simulink model "gm_uz_pmsm_model_nonlinear_vnl"  (R2023a)
settings: Solver=FixedStepAuto  StartTime=0.0  StopTime=0.5  RelTol=1e-3
PreLoadFcn:
  | uz_pmsm_model_init_parameter
PostLoadFcn:
  | % Import the data from Excel for a lookup table
  | FluxMapData = readtable('C:\Users\Philipp\ultrazohm\ultrazohm_sw\ip_cores\uz_pmsm_model\FluxMapData_2023-05-26_13-07-57.csv');
  | % Row indices for lookup table
  | d_current_in_d_axis = FluxMapData(8:27,1:end);
  | % Column indices for lookup table
  | q_current_in_d_axis = FluxMapData(29:48,1:end);
  | % Output values for lookup table
  | d_Flux_d_axis = FluxMapData(50:69,1:end);
undefined symbols (not defined in the file or in its folder): d_current_d_Flux, d_current_q_Flux, Flux_d, Flux_q, friction_coefficient, inertia, k_i_d, k_p_d, k_p_q, L_d, L_q, Ldd, Ldq, Lqd, Lqq, polepair, psi_pm, q_current_d_Flux, q_current_q_Flux, R_1, setpoint_step, simulate_mechanical, simulate_open_loop, static_friction_torque, ts
libraries: hdlmdlgenlib x8, simulink x2, slpidlib x2
(part 1 of 2)
settings Model: Creator=ts  LastModifiedBy=Philipp
settings SolverCC: AlgebraicLoopSolver=TrustRegion  AutoInsertRateTranBlk=on
settings DataIOCC: LimitDataPoints=on  SaveOutput=off  SaveTime=off
settings OptimizationCC: BlockReduction=off  ConditionallyExecuteInputs=off  DefaultParameterBehavior=Inlined  LifeSpan=inf
settings DebuggingCC: AlgebraicLoopMsg=error  InheritedTsInSrcMsg=none  SingleTaskRateTransMsg=error  UnconnectedInputMsg=warning  UnconnectedOutputMsg=warning  UnconnectedLineMsg=warning  AllowSymbolicDim=off  StrictBusMsg=ErrorOnBusTreatedAsVector  SFUnexpectedBacktrackingDiag=warning  SFNoUnconditionalDefaultTransitionDiag=warning  SFExecutionAtInitializationDiag=none  ArithmeticOperatorsInVariantConditions=warning
settings HardwareCC: ProdBitPerPointer=32  ProdBitPerSizeT=32  ProdBitPerPtrDiffT=32  ProdLargestAtomicFloat=None  ProdIntDivRoundTo=Undefined  ProdEndianess=Unspecified  ProdWordSize=32  ProdHWDeviceType=ASIC/FPGA->ASIC/FPGA  ProdEqTarget=off
settings ModelReferenceCC: EnableRefExpFcnMdlSchedulingChecks=on
settings SFSimCC: SimUseLocalCustomCode=off  CustomCodeUndefinedFunction=UseInterfaceOnly
settings RTWCC: RTWUseLocalCustomCode=off  DLArmComputeVersion=19.05
settings CodeAppCC: StateflowObjectComments=on
settings GRTTargetCC: TargetLangStandard=C89/C90 (ANSI)
settings ConfigComp: CovScope=ReferencedModels  CovMetricSettings=dw  CovSaveCumulativeToWorkspaceVar=on  CovSaveSingleToWorkspaceVar=on  CovExternalEMLEnable=off  CovSFcnEnable=off

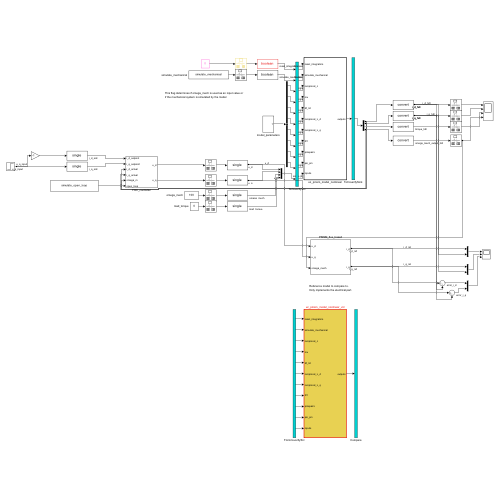
[thumbnail: Simulink's stored preview of the top-level diagram]
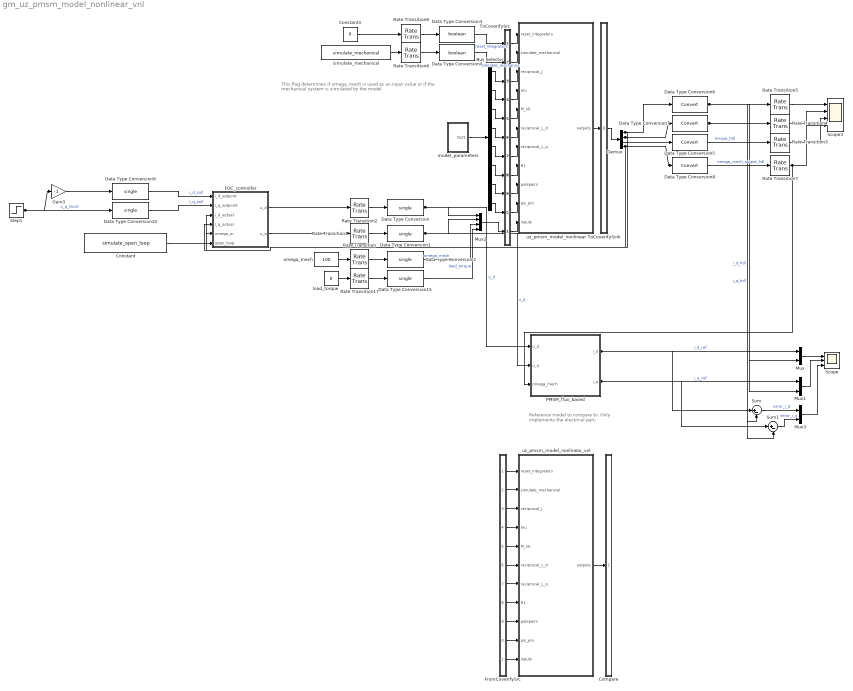
== system gm_uz_pmsm_model_nonlinear_vnl ==
  note: Reference model to compare to.
      | Only implements the electrical part.
  note: This flag determines if omega_mech is used as an input value or
      | if the mechanical system is simulated by the model
  Bus Selector : BusSelector  OutputSignals=1_J,mu,M_R0,1_L_d,1_L_q,R_1,polepair,psi_pm
  Compare : Subsystem
      mask Display: disp('')
  Constant : Constant  Value=simulate_open_loop
  Constant3 : Constant  Value=0
  Data Type Conversion{,1..2,9..10,15} (6 alike) : DataTypeConversion  OutDataTypeStr=single  SaturateOnIntegerOverflow=off  RndMeth=Floor
  Data Type Conversion3 : DataTypeConversion  OutDataTypeStr=boolean  SaturateOnIntegerOverflow=off  RndMeth=Floor
  Data Type Conversion4 : DataTypeConversion  OutDataTypeStr=boolean  SaturateOnIntegerOverflow=off  RndMeth=Floor
  Data Type Conversion{5..8} (4 alike) : DataTypeConversion  SaturateOnIntegerOverflow=off  RndMeth=Floor
  Demux : Demux
  FOC_controller : Subsystem
  FromCoverifySrc : Subsystem
      mask Display: disp('')
  Gain3 : Gain  Gain=-1
  Mux : Mux  Inputs=2
  Mux1 : Mux  Inputs=2
  Mux2 : Mux
  Mux3 : Mux  Inputs=2
  PMSM_flux_based : Subsystem
  Rate Transition{,1..2,6,8,17} (6 alike) : RateTransition  OutPortSampleTime=ts
  Rate Transition{3..5,7} (4 alike) : RateTransition
  Scope : Scope  NumInputPorts=3
  Scope3 : Scope  NumInputPorts=4
  Step1 : Step  Time=0.2  After=setpoint_step
  Sum : Sum  Inputs=|+-
  Sum1 : Sum  Inputs=|+-
  ToCoverifySink : Subsystem
      mask Display: disp('')
  ToCoverifySrc : Subsystem
      mask Display: disp('')
  load_torque : Constant  Value=0
  model_parameters : Subsystem
  omega_mech : Constant  Value=100
  simulate_mechanical : Constant  Value=simulate_mechanical
  uz_pmsm_model_nonlinear : Subsystem  TreatAsAtomicUnit=on
  uz_pmsm_model_nonlinear_vnl : Subsystem  TreatAsAtomicUnit=on
  wires:
  Rate Transition/1 -> Data Type Conversion2/1
  Rate Transition1/1 -> Data Type Conversion1/1
  Rate Transition2/1 -> Data Type Conversion/1
  Data Type Conversion6/1 -> Mux/2, Sum/2, Rate Transition5/1  "i_d_hdl"
  Data Type Conversion7/1 -> Rate Transition4/1, Mux1/2, Sum1/2  "i_q_hdl"
  Data Type Conversion5/1 -> Rate Transition3/1  "torque_hdl"
  Rate Transition4/1 -> Scope3/2
  Rate Transition5/1 -> Scope3/1
  Rate Transition3/1 -> Scope3/3
  Rate Transition6/1 -> Data Type Conversion3/1
  Constant3/1 -> Rate Transition6/1
  Rate Transition8/1 -> Data Type Conversion4/1
  simulate_mechanical/1 -> Rate Transition8/1
  load_torque/1 -> Rate Transition17/1
  Rate Transition17/1 -> Data Type Conversion15/1
  Mux/1 -> Scope/1
  Mux1/1 -> Scope/2
  PMSM_flux_based/2(i_q) -> Mux1/1, Sum1/1  "i_q_ref"
  PMSM_flux_based/1(i_d) -> Mux/1, Sum/1  "i_d_ref"
  Data Type Conversion8/1 -> Rate Transition7/1  "omega_mech_output_hdl"
  Rate Transition7/1 -> PMSM_flux_based/3(omega_mech), Scope3/4
  model_parameters/1(Out1) -> Bus Selector/1
  Sum/1 -> Mux3/1  "error_i_d"
  Sum1/1 -> Mux3/2  "error_i_q"
  Mux3/1 -> Scope/3
  Step1/1 -> Gain3/1, Data Type Conversion10/1  "u_q_input"
  Demux/3 -> Data Type Conversion5/1
  Gain3/1 -> Data Type Conversion9/1
  Demux/1 -> Data Type Conversion6/1, FOC_controller/3(i_d_actual)
  Demux/4 -> Data Type Conversion8/1, FOC_controller/5(omega_m)
  Demux/2 -> Data Type Conversion7/1, FOC_controller/4(i_q_actual)
  Data Type Conversion/1 -> PMSM_flux_based/1(u_d), Mux2/1  "u_d"
  Data Type Conversion1/1 -> PMSM_flux_based/2(u_q), Mux2/2  "u_q"
  Data Type Conversion15/1 -> Mux2/4  "load_torque"
  Data Type Conversion2/1 -> Mux2/3  "omega_mech"
  Data Type Conversion9/1 -> FOC_controller/1(i_d_setpont)  "i_d_soll"
  Data Type Conversion10/1 -> FOC_controller/2(i_q_setpoint)  "i_q_soll"
  FOC_controller/1(u_d) -> Rate Transition2/1
  FOC_controller/2(u_q) -> Rate Transition1/1
  omega_mech/1 -> Rate Transition/1
  Constant/1 -> FOC_controller/6(open_loop)
  ToCoverifySrc/1(out1) -> uz_pmsm_model_nonlinear/1(reset_integrators)
  ToCoverifySrc/2(out2) -> uz_pmsm_model_nonlinear/2(simulate_mechanical)
  ToCoverifySrc/3(out3) -> uz_pmsm_model_nonlinear/3(reciprocal_J)
  ToCoverifySrc/4(out4) -> uz_pmsm_model_nonlinear/4(mu)
  ToCoverifySrc/5(out5) -> uz_pmsm_model_nonlinear/5(M_n0)
  ToCoverifySrc/6(out6) -> uz_pmsm_model_nonlinear/6(reciprocal_L_d)
  ToCoverifySrc/7(out7) -> uz_pmsm_model_nonlinear/7(reciprocal_L_q)
  ToCoverifySrc/8(out8) -> uz_pmsm_model_nonlinear/8(R1)
  ToCoverifySrc/9(out9) -> uz_pmsm_model_nonlinear/9(polepairs)
  ToCoverifySrc/10(out10) -> uz_pmsm_model_nonlinear/10(psi_pm)
  ToCoverifySrc/11(out11) -> uz_pmsm_model_nonlinear/11(inputs)
  uz_pmsm_model_nonlinear/1(outputs) -> ToCoverifySink/1(in1)
  Data Type Conversion3/1 -> ToCoverifySrc/1(in1)  "reset_integrators"
  Data Type Conversion4/1 -> ToCoverifySrc/2(in2)  "simulate_mechanics"
  Bus Selector/1 -> ToCoverifySrc/3(in3)
  Bus Selector/2 -> ToCoverifySrc/4(in4)
  Bus Selector/3 -> ToCoverifySrc/5(in5)
  Bus Selector/4 -> ToCoverifySrc/6(in6)
  Bus Selector/5 -> ToCoverifySrc/7(in7)
  Bus Selector/6 -> ToCoverifySrc/8(in8)
  Bus Selector/7 -> ToCoverifySrc/9(in9)
  Bus Selector/8 -> ToCoverifySrc/10(in10)
  Mux2/1 -> ToCoverifySrc/11(in11)
  ToCoverifySink/1(out1) -> Demux/1
  FromCoverifySrc/1(out1) -> uz_pmsm_model_nonlinear_vnl/1(reset_integrators)
  FromCoverifySrc/2(out2) -> uz_pmsm_model_nonlinear_vnl/2(simulate_mechanical)
  FromCoverifySrc/3(out3) -> uz_pmsm_model_nonlinear_vnl/3(reciprocal_J)
  FromCoverifySrc/4(out4) -> uz_pmsm_model_nonlinear_vnl/4(mu)
  FromCoverifySrc/5(out5) -> uz_pmsm_model_nonlinear_vnl/5(M_n0)
  FromCoverifySrc/6(out6) -> uz_pmsm_model_nonlinear_vnl/6(reciprocal_L_d)
  FromCoverifySrc/7(out7) -> uz_pmsm_model_nonlinear_vnl/7(reciprocal_L_q)
  FromCoverifySrc/8(out8) -> uz_pmsm_model_nonlinear_vnl/8(R1)
  FromCoverifySrc/9(out9) -> uz_pmsm_model_nonlinear_vnl/9(polepairs)
  FromCoverifySrc/10(out10) -> uz_pmsm_model_nonlinear_vnl/10(psi_pm)
  FromCoverifySrc/11(out11) -> uz_pmsm_model_nonlinear_vnl/11(inputs)
  uz_pmsm_model_nonlinear_vnl/1(outputs) -> Compare/1(in1)

== system gm_uz_pmsm_model_nonlinear_vnl/Compare ==
  in1 : Inport
  Assert_outputs : Subsystem  mask{ToleranceValue=1e-07}
      settings: LibrarySourceBlock=hdlmdlgenlib/AssertRelEqIDC
  CleanupScopes : Subsystem
      settings: OpenFcn=|
      | blkName = gcb; %self block
      | idx = regexp(blkName, '/CleanupScopes$', 'once');
      | blkParent = blkName(1:idx-1);
      | blks=find_system(blkParent, 'LookUnderMasks', 'all','blocktype', 'Scope');
      | for itr = 1:length(blks)
      | 	 hScopeCfg = get_param(blks{itr},'ScopeConfiguration');
      | 	 hScopeCfg.Visible = ~ hScopeCfg.Visible;
      | end
      | drawnow;
      mask Display: fprintf(message('hdlcoder:cosim:vnl_dblclick').getString());
  Enable : Subsystem
      settings: OpenFcn=|
      | blkName = gcb;
      | idx = regexp(blkName, '/Enable$', 'once');
      | blkParent = blkName(1:idx-1);
      | blks=find_system(blkParent, 'LookUnderMasks', 'all','blocktype', 'Assertion');
      | e = get_param(blks{1}, 'Enabled');
      | if strcmp(e, 'on'), f= 'off';, else, f = 'on';, end
      | for ii=1:length(blks), set_param(blks{ii}, 'Enabled', f);, end
      | set_param(gcb, 'MaskDisplay',['fprintf(message(''hdlcoder:cosim:vnl_dblclick_assertions'',','''',upper(e),'''',').getString())']);
      mask Display: fprintf(message('hdlcoder:cosim:vnl_dblclick_assertions','OFF').getString());
  pathdelay1 : Delay  DelayLength=1
  wires:
  in1/1 -> pathdelay1/1
  pathdelay1/1 -> Assert_outputs/1(cosim)
  [out1] -> Assert_outputs/2(dut)

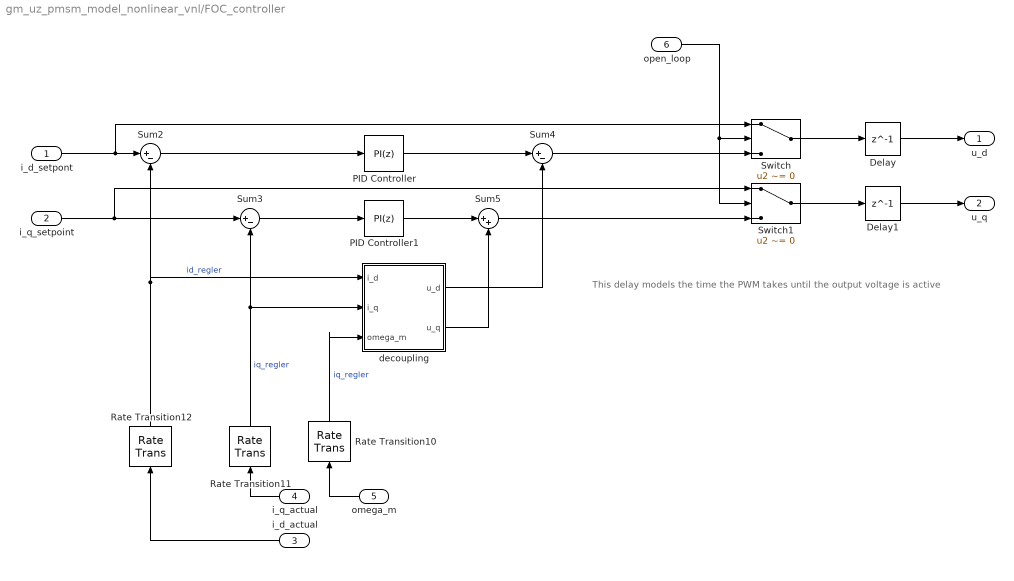
== system gm_uz_pmsm_model_nonlinear_vnl/FOC_controller ==
  note: This delay models the time the PWM takes until the output voltage is active
  i_d_setpont : Inport
  i_q_setpoint : Inport  Port=2
  i_d_actual : Inport  Port=3
  i_q_actual : Inport  Port=4
  omega_m : Inport  Port=5
  open_loop : Inport  Port=6
  Delay : Delay  DelayLength=1
  Delay1 : Delay  DelayLength=1
  PID Controller : slpidlib/PID Controller  Controller=PI  Form=Parallel  TimeDomain=Discrete-time  UseExternalTs=off  SampleTime=-1  IntegratorMethod=Forward Euler  FilterMethod=Forward Euler  ControllerParametersSource=internal  P=k_p_d  I=k_i_d  UseKiTs=off  D=0  N=100  UseFilter=on  TunerSelectOption=Transfer Function Based (PID Tuner App)  InitialConditionSource=internal  InitialConditionForIntegrator=0  InitialConditionForFilter=0  DifferentiatorICPrevScaledInput=0  ExternalReset=none  TrackingMode=off  Kt=1  LimitOutput=off  SatLimitsSource=internal  UpperSaturationLimit=inf  LowerSaturationLimit=-inf  LinearizeAsGain=on  AntiWindupMode=none  Kb=1  LimitIntegrator=off  UpperIntegratorSaturationLimit=inf  LowerIntegratorSaturationLimit=-inf  POutMin=[]  POutMax=[]  IOutMin=[]  IOutMax=[]  DOutMin=[]  DOutMax=[]  NOutMin=[]  NOutMax=[]  SumOutMin=[]  SumOutMax=[]  SaturationOutMin=[]  SaturationOutMax=[]  PParamMin=[]  PParamMax=[]  IParamMin=[]  IParamMax=[]  DParamMin=[]  DParamMax=[]  NParamMin=[]  NParamMax=[]  KbParamMin=[]  KbParamMax=[]  KtParamMin=[]  KtParamMax=[]  KbOutMin=[]  KbOutMax=[]  KtOutMin=[]  KtOutMax=[]  IntegratorOutMin=[]  IntegratorOutMax=[]  FilterOutMin=[]  FilterOutMax=[]  SumI1OutMin=[]  SumI1OutMax=[]  SumI2OutMin=[]  SumI2OutMax=[]  SumI3OutMin=[]  SumI3OutMax=[]  SumI4OutMin=[]  SumI4OutMax=[]  SumDOutMin=[]  SumDOutMax=[]  DifferentiatorOutMin=[]  DifferentiatorOutMax=[]  FilterDiffOutCoefMin=[]  FilterDiffOutCoefMax=[]  ReciprocalOutMin=[]  ReciprocalOutMax=[]  SumDenOutMin=[]  SumDenOutMax=[]  SumNumOutMin=[]  SumNumOutMax=[]  DivideOutMin=[]  DivideOutMax=[]  UdiffTsProdOutMin=[]  UdiffTsProdOutMax=[]  NTsProdOutMin=[]  NTsProdOutMax=[]  UintegralTsProdOutMin=[]  UintegralTsProdOutMax=[]  UngainTsProdOutMin=[]  UngainTsProdOutMax=[]  ClampingZeroOutDataTypeStr=Inherit: Inherit via back propagation  ClampingZeroOutMin=[]  ClampingZeroOutMax=[]  FilterDenConstantOutDataTypeStr=Inherit: Inherit via back propagation  FilterDenConstantOutMin=[]  FilterDenConstantOutMax=[]  PCopyOutDataTypeStr=Inherit: Inherit via back propagation  PCopyOutMin=[]  PCopyOutMax=[]  NCopyOutDataTypeStr=Inherit: Inherit via back propagation  NCopyOutMin=[]  NCopyOutMax=[]  IntegratorContinuousStateAttributes=''  IntegratorStateMustResolveToSignalObject=off  IntegratorRTWStateStorageClass=Auto  FilterContinuousStateAttributes=''  FilterStateMustResolveToSignalObject=off  FilterRTWStateStorageClass=Auto  ParallelPVariant=InternalParameters  IdealPVariant=Disabled  IVariant=InternalParameters  DVariant=Disabled  IntegratorVariant=Discrete  SatVariant=Disabled  AWVariant=Passthrough  PCopyVariant=Disabled  TRVariant=Disabled  FdbkBlocksVariant=Forward  IdealPFdbkVariant=Disabled  SatFdbkVariant=Disabled  DerivativeFilterVariant=Disabled  NVariant=Disabled  NCopyVariant=Disabled_SignalSpec  FilterICVariant=Disabled  IntegratorICVariant=InternalICs  ExternalResetVariant=Disabled  TRSumVariant=Passthrough  SumFdbkVariant=Disabled  SumVariant=Sum_PI  TsampFilterVariant=InternalTs  TsampNgainVariant=Passthrough  TsampIntegralVariant=Disabled_SignalSpec  ExternalSaturationOutDataTypeStr=Inherit: Same as second input
  PID Controller1 : slpidlib/PID Controller  Controller=PI  Form=Parallel  TimeDomain=Discrete-time  UseExternalTs=off  SampleTime=-1  IntegratorMethod=Forward Euler  FilterMethod=Forward Euler  ControllerParametersSource=internal  P=k_p_q  I=k_i_d  UseKiTs=off  D=0  N=100  UseFilter=on  TunerSelectOption=Transfer Function Based (PID Tuner App)  InitialConditionSource=internal  InitialConditionForIntegrator=0  InitialConditionForFilter=0  DifferentiatorICPrevScaledInput=0  ExternalReset=none  TrackingMode=off  Kt=1  LimitOutput=off  SatLimitsSource=internal  UpperSaturationLimit=inf  LowerSaturationLimit=-inf  LinearizeAsGain=on  AntiWindupMode=none  Kb=1  LimitIntegrator=off  UpperIntegratorSaturationLimit=inf  LowerIntegratorSaturationLimit=-inf  POutMin=[]  POutMax=[]  IOutMin=[]  IOutMax=[]  DOutMin=[]  DOutMax=[]  NOutMin=[]  NOutMax=[]  SumOutMin=[]  SumOutMax=[]  SaturationOutMin=[]  SaturationOutMax=[]  PParamMin=[]  PParamMax=[]  IParamMin=[]  IParamMax=[]  DParamMin=[]  DParamMax=[]  NParamMin=[]  NParamMax=[]  KbParamMin=[]  KbParamMax=[]  KtParamMin=[]  KtParamMax=[]  KbOutMin=[]  KbOutMax=[]  KtOutMin=[]  KtOutMax=[]  IntegratorOutMin=[]  IntegratorOutMax=[]  FilterOutMin=[]  FilterOutMax=[]  SumI1OutMin=[]  SumI1OutMax=[]  SumI2OutMin=[]  SumI2OutMax=[]  SumI3OutMin=[]  SumI3OutMax=[]  SumI4OutMin=[]  SumI4OutMax=[]  SumDOutMin=[]  SumDOutMax=[]  DifferentiatorOutMin=[]  DifferentiatorOutMax=[]  FilterDiffOutCoefMin=[]  FilterDiffOutCoefMax=[]  ReciprocalOutMin=[]  ReciprocalOutMax=[]  SumDenOutMin=[]  SumDenOutMax=[]  SumNumOutMin=[]  SumNumOutMax=[]  DivideOutMin=[]  DivideOutMax=[]  UdiffTsProdOutMin=[]  UdiffTsProdOutMax=[]  NTsProdOutMin=[]  NTsProdOutMax=[]  UintegralTsProdOutMin=[]  UintegralTsProdOutMax=[]  UngainTsProdOutMin=[]  UngainTsProdOutMax=[]  ClampingZeroOutDataTypeStr=Inherit: Inherit via back propagation  ClampingZeroOutMin=[]  ClampingZeroOutMax=[]  FilterDenConstantOutDataTypeStr=Inherit: Inherit via back propagation  FilterDenConstantOutMin=[]  FilterDenConstantOutMax=[]  PCopyOutDataTypeStr=Inherit: Inherit via back propagation  PCopyOutMin=[]  PCopyOutMax=[]  NCopyOutDataTypeStr=Inherit: Inherit via back propagation  NCopyOutMin=[]  NCopyOutMax=[]  IntegratorContinuousStateAttributes=''  IntegratorStateMustResolveToSignalObject=off  IntegratorRTWStateStorageClass=Auto  FilterContinuousStateAttributes=''  FilterStateMustResolveToSignalObject=off  FilterRTWStateStorageClass=Auto  ParallelPVariant=InternalParameters  IdealPVariant=Disabled  IVariant=InternalParameters  DVariant=Disabled  IntegratorVariant=Discrete  SatVariant=Disabled  AWVariant=Passthrough  PCopyVariant=Disabled  TRVariant=Disabled  FdbkBlocksVariant=Forward  IdealPFdbkVariant=Disabled  SatFdbkVariant=Disabled  DerivativeFilterVariant=Disabled  NVariant=Disabled  NCopyVariant=Disabled_SignalSpec  FilterICVariant=Disabled  IntegratorICVariant=InternalICs  ExternalResetVariant=Disabled  TRSumVariant=Passthrough  SumFdbkVariant=Disabled  SumVariant=Sum_PI  TsampFilterVariant=InternalTs  TsampNgainVariant=Passthrough  TsampIntegralVariant=Disabled_SignalSpec  ExternalSaturationOutDataTypeStr=Inherit: Same as second input
  Rate Transition10 : RateTransition  OutPortSampleTime=ts_regler
  Rate Transition11 : RateTransition  OutPortSampleTime=ts_regler
  Rate Transition12 : RateTransition  OutPortSampleTime=ts_regler
  Sum2 : Sum  Inputs=|+-
  Sum3 : Sum  Inputs=|+-
  Sum4 : Sum  Inputs=|+-
  Sum5 : Sum  Inputs=|++
  Switch : Switch  Criteria=u2 ~= 0  SaturateOnIntegerOverflow=off  InputSameDT=off
  Switch1 : Switch  Criteria=u2 ~= 0  SaturateOnIntegerOverflow=off  InputSameDT=off
  decoupling : Subsystem
  u_d : Outport
  u_q : Outport  Port=2
  wires:
  PID Controller/1 -> Sum4/1
  PID Controller1/1 -> Sum5/1
  Sum4/1 -> Switch/3
  i_d_actual/1 -> Rate Transition12/1
  i_d_setpont/1 -> Switch/1, Sum2/1
  Sum2/1 -> PID Controller/1
  Sum5/1 -> Switch1/3
  omega_m/1 -> Rate Transition10/1
  Sum3/1 -> PID Controller1/1
  i_q_actual/1 -> Rate Transition11/1
  Rate Transition12/1 -> decoupling/1(i_d), Sum2/2  "id_regler"
  Rate Transition11/1 -> decoupling/2(i_q), Sum3/2  "iq_regler"
  i_q_setpoint/1 -> Switch1/1, Sum3/1
  open_loop/1 -> Switch1/2, Switch/2
  Rate Transition10/1 -> decoupling/3(omega_m)  "iq_regler"
  decoupling/1(u_d) -> Sum4/2
  decoupling/2(u_q) -> Sum5/2
  Switch/1 -> Delay/1
  Switch1/1 -> Delay1/1
  Delay/1 -> u_d/1
  Delay1/1 -> u_q/1

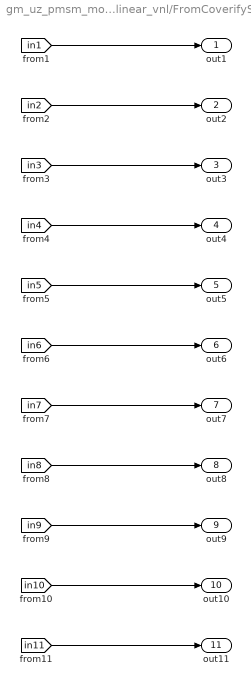
== system gm_uz_pmsm_model_nonlinear_vnl/FromCoverifySrc ==
  out1 : Outport
  out2 : Outport  Port=2
  out3 : Outport  Port=3
  out4 : Outport  Port=4
  out5 : Outport  Port=5
  out6 : Outport  Port=6
  out7 : Outport  Port=7
  out8 : Outport  Port=8
  out9 : Outport  Port=9
  out10 : Outport  Port=10
  out11 : Outport  Port=11
  wires:
  [in1] -> out1/1
  [in2] -> out2/1
  [in3] -> out3/1
  [in4] -> out4/1
  [in5] -> out5/1
  [in6] -> out6/1
  [in7] -> out7/1
  [in8] -> out8/1
  [in9] -> out9/1
  [in10] -> out10/1
  [in11] -> out11/1

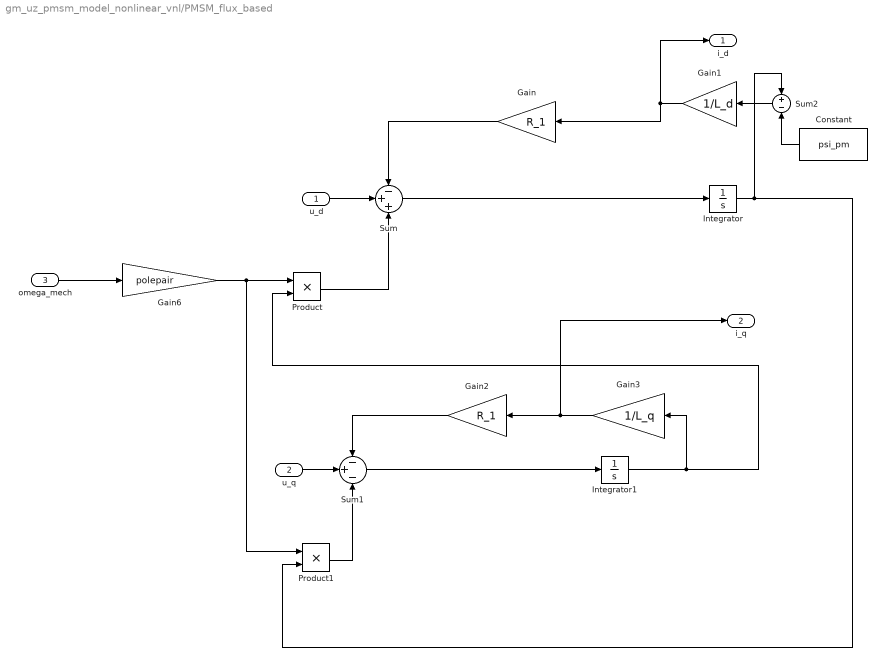
== system gm_uz_pmsm_model_nonlinear_vnl/PMSM_flux_based ==
  u_d : Inport
  u_q : Inport  Port=2
  omega_mech : Inport  Port=3
  Constant : Constant  Value=psi_pm
  Gain : Gain  Gain=R_1
  Gain1 : Gain  Gain=1/L_d
  Gain2 : Gain  Gain=R_1
  Gain3 : Gain  Gain=1/L_q
  Gain6 : Gain  Gain=polepair
  Integrator : Integrator
  Integrator1 : Integrator
  Product : Product
  Product1 : Product
  Sum : Sum  Inputs=-++
  Sum1 : Sum  Inputs=-+-
  Sum2 : Sum  Inputs=+-
  i_d : Outport
  i_q : Outport  Port=2
  wires:
  u_d/1 -> Sum/2
  u_q/1 -> Sum1/2
  Sum/1 -> Integrator/1
  Gain/1 -> Sum/1
  Integrator/1 -> Product1/2, Sum2/1
  Constant/1 -> Sum2/2
  Sum2/1 -> Gain1/1
  Gain1/1 -> Gain/1, i_d/1
  Gain6/1 -> Product1/1, Product/1
  Product/1 -> Sum/3
  Integrator1/1 -> Gain3/1, Product/2
  Product1/1 -> Sum1/3
  Sum1/1 -> Integrator1/1
  Gain2/1 -> Sum1/1
  Gain3/1 -> i_q/1, Gain2/1
  omega_mech/1 -> Gain6/1

== system gm_uz_pmsm_model_nonlinear_vnl/ToCoverifySink ==
  in1 : Inport
  out1 : Outport
  tag scope: out1=global
  wires:
  in1/1 -> out1/1, [out1]

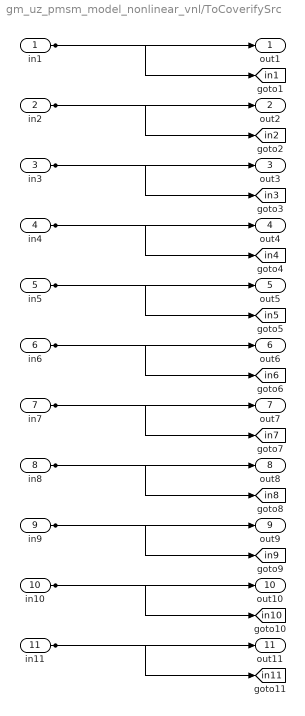
== system gm_uz_pmsm_model_nonlinear_vnl/ToCoverifySrc ==
  in1 : Inport
  in2 : Inport  Port=2
  in3 : Inport  Port=3
  in4 : Inport  Port=4
  in5 : Inport  Port=5
  in6 : Inport  Port=6
  in7 : Inport  Port=7
  in8 : Inport  Port=8
  in9 : Inport  Port=9
  in10 : Inport  Port=10
  in11 : Inport  Port=11
  out1 : Outport
  out2 : Outport  Port=2
  out3 : Outport  Port=3
  out4 : Outport  Port=4
  out5 : Outport  Port=5
  out6 : Outport  Port=6
  out7 : Outport  Port=7
  out8 : Outport  Port=8
  out9 : Outport  Port=9
  out10 : Outport  Port=10
  out11 : Outport  Port=11
  tag scope: in10=global, in11=global, in1=global, in2=global, in3=global, in4=global, in5=global, in6=global, in7=global, in8=global, in9=global
  wires:
  in1/1 -> out1/1, [in1]
  in2/1 -> out2/1, [in2]
  in3/1 -> out3/1, [in3]
  in4/1 -> out4/1, [in4]
  in5/1 -> out5/1, [in5]
  in6/1 -> out6/1, [in6]
  in7/1 -> out7/1, [in7]
  in8/1 -> out8/1, [in8]
  in9/1 -> out9/1, [in9]
  in10/1 -> out10/1, [in10]
  in11/1 -> out11/1, [in11]

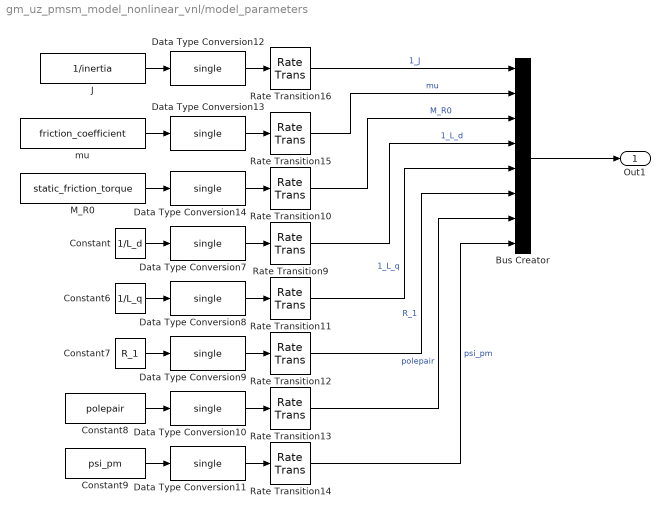
== system gm_uz_pmsm_model_nonlinear_vnl/model_parameters ==
  Bus Creator : BusCreator  Inputs=8
  Constant : Constant  Value=1/L_d
  Constant6 : Constant  Value=1/L_q
  Constant7 : Constant  Value=R_1
  Constant8 : Constant  Value=polepair
  Constant9 : Constant  Value=psi_pm
  Data Type Conversion{7..14} (8 alike) : DataTypeConversion  OutDataTypeStr=single  SaturateOnIntegerOverflow=off  RndMeth=Floor
  J : Constant  Value=1/inertia
  M_R0 : Constant  Value=static_friction_torque
  Rate Transition{9..16} (8 alike) : RateTransition  OutPortSampleTime=ts
  mu : Constant  Value=friction_coefficient
  Out1 : Outport
  wires:
  Data Type Conversion12/1 -> Rate Transition16/1
  Data Type Conversion7/1 -> Rate Transition9/1
  Rate Transition10/1 -> Bus Creator/3  "M_R0"
  Rate Transition14/1 -> Bus Creator/8  "psi_pm"
  Data Type Conversion14/1 -> Rate Transition10/1
  Rate Transition12/1 -> Bus Creator/6  "R_1"
  Rate Transition16/1 -> Bus Creator/1  "1_J"
  Rate Transition13/1 -> Bus Creator/7  "polepair"
  Bus Creator/1 -> Out1/1
  Data Type Conversion11/1 -> Rate Transition14/1
  Constant8/1 -> Data Type Conversion10/1
  Data Type Conversion9/1 -> Rate Transition12/1
  Rate Transition15/1 -> Bus Creator/2  "mu"
  Constant6/1 -> Data Type Conversion8/1
  Rate Transition9/1 -> Bus Creator/4  "1_L_d"
  J/1 -> Data Type Conversion12/1
  Data Type Conversion8/1 -> Rate Transition11/1
  Data Type Conversion10/1 -> Rate Transition13/1
  mu/1 -> Data Type Conversion13/1
  M_R0/1 -> Data Type Conversion14/1
  Rate Transition11/1 -> Bus Creator/5  "1_L_q"
  Data Type Conversion13/1 -> Rate Transition15/1
  Constant7/1 -> Data Type Conversion9/1
  Constant9/1 -> Data Type Conversion11/1
  Constant/1 -> Data Type Conversion7/1

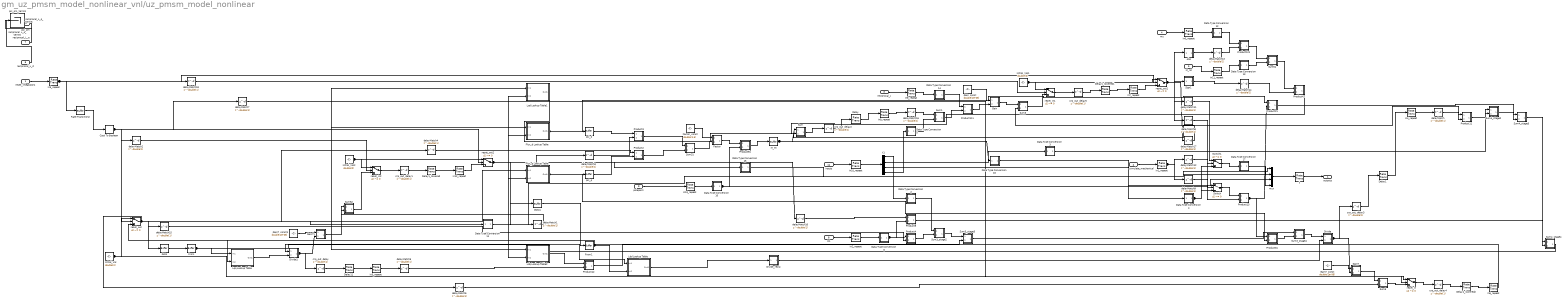
== system gm_uz_pmsm_model_nonlinear_vnl/uz_pmsm_model_nonlinear ==
  reset_integrators : Inport  OutDataTypeStr=boolean  PortDimensions=1  SampleTime=2e-06
  simulate_mechanical : Inport  Port=2  OutDataTypeStr=boolean  PortDimensions=1  SampleTime=2e-06
  reciprocal_J : Inport  Port=3  OutDataTypeStr=single  PortDimensions=1  SampleTime=2e-06
  mu : Inport  Port=4  OutDataTypeStr=single  PortDimensions=1  SampleTime=2e-06
  M_n0 : Inport  Port=5  OutDataTypeStr=single  PortDimensions=1  SampleTime=2e-06
  reciprocal_L_d : Inport  Port=6  OutDataTypeStr=single  PortDimensions=1  SampleTime=2e-06
  reciprocal_L_q : Inport  Port=7  OutDataTypeStr=single  PortDimensions=1  SampleTime=2e-06
  R1 : Inport  Port=8  OutDataTypeStr=single  PortDimensions=1  SampleTime=2e-06
  polepairs : Inport  Port=9  OutDataTypeStr=single  PortDimensions=1  SampleTime=2e-06
  psi_pm : Inport  Port=10  OutDataTypeStr=single  PortDimensions=1  SampleTime=2e-06
  inputs : Inport  Port=11  OutDataTypeStr=single  PortDimensions=[4]  SampleTime=2e-06
  Abs : Subsystem
      mask Display: disp('NFP\nabs');
  Cast To Boolean : DataTypeConversion  OutDataTypeStr=boolean
  Data Type Conversion10 : Subsystem
      mask Display: disp('NFP\nconv');
  Data Type Conversion11 : Subsystem
      mask Display: disp('NFP\nconv');
  Data Type Conversion12 : Subsystem
      mask Display: disp('NFP\nconv');
  Data Type Conversion13 : Subsystem
      mask Display: disp('NFP\nconv');
  Data Type Conversion14 : Subsystem
      mask Display: disp('NFP\nconv');
  Data Type Conversion15 : Subsystem
      mask Display: disp('NFP\nconv');
  Data Type Conversion16 : Subsystem
      mask Display: disp('NFP\nconv');
  Data Type Conversion17 : Subsystem
      mask Display: disp('NFP\nconv');
  Data Type Conversion2 : Subsystem
      mask Display: disp('NFP\nconv');
  Data Type Conversion3 : Subsystem
      mask Display: disp('NFP\nconv');
  Data Type Conversion4 : Subsystem
      mask Display: disp('NFP\nconv');
  Data Type Conversion5 : Subsystem
      mask Display: disp('NFP\nconv');
  Data Type Conversion6 : Subsystem
      mask Display: disp('NFP\nconv');
  Delay : RateTransition  OutPortSampleTimeOpt=Multiple of input port sample time  OutPortSampleTimeMultiple=200
  Delay1 : RateTransition  OutPortSampleTimeOpt=Multiple of input port sample time  OutPortSampleTimeMultiple=200
  Delay11 : RateTransition  OutPortSampleTimeOpt=Multiple of input port sample time  OutPortSampleTimeMultiple=200
  Delay1_lowered : RateTransition  OutPortSampleTimeOpt=Multiple of input port sample time  OutPortSampleTimeMultiple=200
  Delay1_lowered1 : RateTransition  OutPortSampleTimeOpt=Multiple of input port sample time  OutPortSampleTimeMultiple=200
  Delay1_lowered2 : RateTransition  OutPortSampleTimeOpt=Multiple of input port sample time  OutPortSampleTimeMultiple=200
  Divide : Subsystem
      mask Display: disp('NFP\nmul');
  Divide1 : Subsystem
      mask Display: disp('NFP\nmul');
  Divide_recip : Subsystem
      mask Display: disp('NFP\nmath');
  Factor : Subsystem
      mask Display: disp('NFP\nmul');
  Factor_const : Constant  Value=double(1.5)  OutDataTypeStr=double  SampleTime=1e-08
  Flux_d Lookup Table : Subsystem
  Flux_q Lookup Table : Subsystem
  From : hdlmdlgenlib/Buffer
  From1 : hdlmdlgenlib/Buffer
  Gain : Subsystem
      mask Display: disp('NFP\nmul');
  Gain7 : Subsystem
      mask Display: disp('NFP\nmul');
  Gain71 : Subsystem
      mask Display: disp('NFP\nmul');
  Gain7_const : Constant  Value=double(2e-06)  OutDataTypeStr=double  SampleTime=1e-08
  Gain7_const1 : Constant  Value=double(2e-06)  OutDataTypeStr=double  SampleTime=1e-08
  Gain_const : Constant  Value=double(2e-06)  OutDataTypeStr=double  SampleTime=1e-08
  Goto : hdlmdlgenlib/Buffer
  Goto1 : hdlmdlgenlib/Buffer
  Initial_Val : Constant  Value=double(0)  OutDataTypeStr=double  SampleTime=1e-08
  Initial_Val1 : Constant  Value=double(0)  OutDataTypeStr=double  SampleTime=1e-08
  Initial_Val2 : Constant  Value=double(0)  OutDataTypeStr=double  SampleTime=1e-08
  Ldd Lookup Table : Subsystem
  Ldq Lookup Table2 : Subsystem
  Lqd Lookup Table1 : Subsystem
  Lqq Lookup Table : Subsystem
  M_Mi : hdlmdlgenlib/Buffer
  Product11 : Subsystem
      mask Display: disp('NFP\nmul');
  Product111 : Subsystem
      mask Display: disp('NFP\nmul');
  Product12 : Subsystem
      mask Display: disp('NFP\nmul');
  Product121 : Subsystem
      mask Display: disp('NFP\nmul');
  Product13 : Subsystem
      mask Display: disp('NFP\nmul');
  Product2 : Subsystem
      mask Display: disp('NFP\nmul');
  Product21 : Subsystem
      mask Display: disp('NFP\nmul');
  Product3 : Subsystem
      mask Display: disp('NFP\nmul');
  Product31 : Subsystem
      mask Display: disp('NFP\nmul');
  Product4 : Subsystem
      mask Display: disp('NFP\nmul');
  Product41 : Subsystem
      mask Display: disp('NFP\nmul');
  Product9 : Subsystem
      mask Display: disp('NFP\nmul');
  Product91 : Subsystem
      mask Display: disp('NFP\nmul');
  Rate Transition2 : hdlmdlgenlib/Buffer
  Sign1 : Subsystem
      mask Display: disp('NFP\nsignum');
  Sum : Subsystem
      mask Display: disp('NFP\nadd');
  Sum1 : Subsystem
      mask Display: disp('NFP\nadd');
  Sum3 : Subsystem
      mask Display: disp('NFP\nadd');
  Sum31 : Subsystem
      mask Display: disp('NFP\nadd');
  Sum3_stage2 : Subsystem
      mask Display: disp('NFP\nadd');
  Sum3_stage3 : Subsystem
      mask Display: disp('NFP\nadd');
  Sum3_stage4 : Subsystem
      mask Display: disp('NFP\nadd');
  Sum4_stage2 : Subsystem
      mask Display: disp('NFP\nadd');
  Sum4_stage3 : Subsystem
      mask Display: disp('NFP\nadd');
  Sum4_stage4 : Subsystem
      mask Display: disp('NFP\nadd');
  Sum5 : Subsystem
      mask Display: disp('NFP\nadd');
  Sum51 : Subsystem
      mask Display: disp('NFP\nadd');
  Sum52 : Subsystem
      mask Display: disp('NFP\nadd');
  Switch : Switch  Criteria=u2 ~= 0  Threshold=double(0)  OutDataTypeStr=double  SampleTime=1e-08  SaturateOnIntegerOverflow=off  InputSameDT=off
  Switch1 : Switch  Criteria=u2 ~= 0  Threshold=double(0)  OutDataTypeStr=double  SampleTime=1e-08  SaturateOnIntegerOverflow=off  InputSameDT=off
  crp_out_delay{,1..5} (6 alike) : Delay  DelayLength=double(1)  InitialCondition=0  SampleTime=1e-08
  delayMatch{,1..18} (19 alike) : Delay  DelayLength=double(1)  InitialCondition=0  SampleTime=1e-08
  in0_repeat : RateTransition  Integrity=off  Deterministic=off  OutPortSampleTimeOpt=Multiple of input port sample time  OutPortSampleTimeMultiple=1/200
  in10_repeat : RateTransition  Integrity=off  Deterministic=off  OutPortSampleTimeOpt=Multiple of input port sample time  OutPortSampleTimeMultiple=1/200
  in11_repeat : RateTransition  Integrity=off  Deterministic=off  OutPortSampleTimeOpt=Multiple of input port sample time  OutPortSampleTimeMultiple=1/200
  in12_repeat : RateTransition  Integrity=off  Deterministic=off  OutPortSampleTimeOpt=Multiple of input port sample time  OutPortSampleTimeMultiple=1/200
  in13_repeat : RateTransition  Integrity=off  Deterministic=off  OutPortSampleTimeOpt=Multiple of input port sample time  OutPortSampleTimeMultiple=1/200
  in1_repeat : RateTransition  Integrity=off  Deterministic=off  OutPortSampleTimeOpt=Multiple of input port sample time  OutPortSampleTimeMultiple=1/200
  in2_repeat : RateTransition  Integrity=off  Deterministic=off  OutPortSampleTimeOpt=Multiple of input port sample time  OutPortSampleTimeMultiple=1/200
  in3_repeat : RateTransition  Integrity=off  Deterministic=off  OutPortSampleTimeOpt=Multiple of input port sample time  OutPortSampleTimeMultiple=1/200
  in4_repeat : RateTransition  Integrity=off  Deterministic=off  OutPortSampleTimeOpt=Multiple of input port sample time  OutPortSampleTimeMultiple=1/200
  in5_repeat : RateTransition  Integrity=off  Deterministic=off  OutPortSampleTimeOpt=Multiple of input port sample time  OutPortSampleTimeMultiple=1/200
  in6_repeat : RateTransition  Integrity=off  Deterministic=off  OutPortSampleTimeOpt=Multiple of input port sample time  OutPortSampleTimeMultiple=1/200
  in7_repeat : RateTransition  Integrity=off  Deterministic=off  OutPortSampleTimeOpt=Multiple of input port sample time  OutPortSampleTimeMultiple=1/200
  in8_repeat : RateTransition  Integrity=off  Deterministic=off  OutPortSampleTimeOpt=Multiple of input port sample time  OutPortSampleTimeMultiple=1/200
  in9_repeat : RateTransition  Integrity=off  Deterministic=off  OutPortSampleTimeOpt=Multiple of input port sample time  OutPortSampleTimeMultiple=1/200
  mux : Mux
  psi_d : hdlmdlgenlib/Buffer
  psi_pm_term9 : Terminator
  psi_q : hdlmdlgenlib/Buffer
  reciprocal_L_d_term5 : Terminator
  reciprocal_L_q_term6 : Terminator
  reset_in : Switch  Criteria=u2 ~= 0  Threshold=double(0)  OutDataTypeStr=double  SampleTime=1e-08  SaturateOnIntegerOverflow=off  InputSameDT=off
  reset_in1 : Switch  Criteria=u2 ~= 0  Threshold=double(0)  OutDataTypeStr=double  SampleTime=1e-08  SaturateOnIntegerOverflow=off  InputSameDT=off
  reset_in2 : Switch  Criteria=u2 ~= 0  Threshold=double(0)  OutDataTypeStr=double  SampleTime=1e-08  SaturateOnIntegerOverflow=off  InputSameDT=off
  reset_out : Switch  Criteria=u2 ~= 0  Threshold=double(0)  OutDataTypeStr=double  SampleTime=1e-08  SaturateOnIntegerOverflow=off  InputSameDT=off
  reset_out1 : Switch  Criteria=u2 ~= 0  Threshold=double(0)  OutDataTypeStr=double  SampleTime=1e-08  SaturateOnIntegerOverflow=off  InputSameDT=off
  reset_out2 : Switch  Criteria=u2 ~= 0  Threshold=double(0)  OutDataTypeStr=double  SampleTime=1e-08  SaturateOnIntegerOverflow=off  InputSameDT=off
  t : RateTransition  OutPortSampleTimeOpt=Multiple of input port sample time  OutPortSampleTimeMultiple=200
  t1 : Demux
  outputs : Outport  SampleTime=2e-06
  wires:
  reset_out1/1 -> delayMatch8/1, delayMatch11/1, Sign1/1(In1), Abs/1(In1), delayMatch17/1
  delayMatch7/1 -> reset_in/2
  delayMatch6/1 -> Sum5/2(In2)
  delayMatch2/1 -> reset_in2/2
  delayMatch1/1 -> Sum52/2(In2)
  delayMatch12/1 -> Switch1/2
  delayMatch11/1 -> Switch1/1
  Gain71/1(Out1) -> Sum52/1(In1)
  Gain/1(Out1) -> Sum3/1(In1)
  Gain7/1(Out1) -> Sum5/1(In1)
  Data Type Conversion10/1(Out1) -> Product91/2(In2), Product13/2(In2)
  Product13/1(Out1) -> Product31/1(In1), Product21/2(In2)
  Sum4_stage4/1(Out1) -> Divide1/1(In1)
  Sum4_stage3/1(Out1) -> Sum4_stage4/1(In1)
  Sum4_stage2/1(Out1) -> Sum4_stage3/1(In1)
  Sum52/1(Out1) -> reset_in2/3
  Data Type Conversion11/1(Out1) -> mux/1
  Product2/1(Out1) -> Sum31/2(In2)
  Sum31/1(Out1) -> Factor/2(In2)
  Sum/1(Out1) -> crp_out_delay2/1
  Product41/1(Out1) -> Sum/2(In2)
  Sum51/1(Out1) -> Product41/1(In1)
  Data Type Conversion13/1(Out1) -> Sum51/2(In2)
  Product121/1(Out1) -> Sum51/1(In1)
  Abs/1(Out1) -> delayMatch13/1
  Sign1/1(Out1) -> delayMatch14/1
  Sum1/1(Out1) -> Product111/2(In2)
  Product111/1(Out1) -> Gain/2(In2)
  Data Type Conversion14/1(Out1) -> Product111/1(In1)
  Sum3/1(Out1) -> reset_in1/3
  Sum3_stage4/1(Out1) -> Divide/1(In1)
  Sum3_stage3/1(Out1) -> Sum3_stage4/1(In1)
  Sum3_stage2/1(Out1) -> Sum3_stage3/1(In1)
  Divide_recip/1(Out1) -> Divide/2(In2)
  Sum5/1(Out1) -> reset_in/3
  Product11/1(Out1) -> Sum4_stage2/2(In2)
  Product12/1(Out1) -> Sum3_stage3/2(In2)
  Product3/1(Out1) -> Sum31/1(In1)
  Product4/1(Out1) -> Sum3_stage2/2(In2)
  Data Type Conversion6/1(Out1) -> Product9/2(In2), Product4/1(In1)
  Product9/1(Out1) -> Sum4_stage4/2(In2)
  Data Type Conversion12/1(Out1) -> Product121/1(In1)
  Cast To Boolean/1 -> reset_out/2, reset_out2/2, delayMatch2/1, delayMatch7/1
  reset_out/1 -> delayMatch4/1, Data Type Conversion11/1(In1), Lqd Lookup Table1/1(In1), Ldq Lookup Table2/1(In1), Flux_q Lookup Table/1(In1), Flux_d Lookup Table/1(In1), Goto/1, delayMatch15/1, delayMatch6/1
  reset_out2/1 -> delayMatch3/1, Data Type Conversion15/1(In1), Lqd Lookup Table1/2(In2), Ldq Lookup Table2/2(In2), Flux_q Lookup Table/2(In2), Flux_d Lookup Table/2(In2), Goto1/1, delayMatch10/1, delayMatch1/1
  delayMatch16/1 -> Sum1/1(In1)
  delayMatch18/1 -> reset_in1/2
  delayMatch9/1 -> Switch/2
  Gain7_const1/1 -> Gain71/1(In1)
  Factor_const/1 -> Factor/1(In1)
  Gain_const/1 -> Gain/1(In1)
  Gain7_const/1 -> Gain7/1(In1)
  delayMatch/1 -> Product11/1(In1)
  delayMatch5/1 -> Product12/2(In2)
  Product21/1(Out1) -> Sum4_stage3/2(In2)
  Divide1/1(Out1) -> crp_out_delay/1, Gain71/2(In2)
  reset_in2/1 -> crp_out_delay1/1
  Initial_Val2/1 -> reset_in2/1, reset_out2/1
  delayMatch10/1 -> Product9/1(In1)
  delayMatch3/1 -> Product3/2(In2)
  Data Type Conversion15/1(Out1) -> mux/2
  delayMatch4/1 -> Product2/1(In1)
  Factor/1(Out1) -> Product91/1(In1)
  Product91/1(Out1) -> M_Mi/1
  M_Mi/1 -> Data Type Conversion16/1(In1), Sum/1(In1)
  delayMatch13/1 -> Product121/2(In2)
  delayMatch14/1 -> Product41/2(In2)
  delayMatch8/1 -> Switch/1
  Switch/1 -> Product13/1(In1)
  Data Type Conversion4/1(Out1) -> Switch1/3, Switch/3
  t1/4 -> Data Type Conversion5/1(In1)
  t1/3 -> Data Type Conversion4/1(In1)
  t1/2 -> Data Type Conversion3/1(In1)
  t1/1 -> Data Type Conversion2/1(In1)
  Data Type Conversion5/1(Out1) -> Sum1/2(In2)
  reset_in1/1 -> crp_out_delay5/1
  Initial_Val1/1 -> reset_in1/1, reset_out1/1
  delayMatch17/1 -> Sum3/2(In2)
  Data Type Conversion3/1(Out1) -> Sum4_stage2/1(In1)
  Data Type Conversion2/1(Out1) -> Sum3_stage2/1(In1)
  Divide/1(Out1) -> crp_out_delay3/1, Gain7/2(In2)
  reset_in/1 -> crp_out_delay4/1
  Initial_Val/1 -> reset_in/1, reset_out/1
  Rate Transition2/1 -> Cast To Boolean/1
  delayMatch15/1 -> Product4/2(In2)
  Lqd Lookup Table1/1(Out1) -> Product11/2(In2)
  Ldq Lookup Table2/1(Out1) -> Product12/1(In1)
  Flux_q Lookup Table/1(Out1) -> psi_q/1, Product31/2(In2)
  Product31/1(Out1) -> Sum3_stage4/2(In2)
  psi_q/1 -> Product2/2(In2)
  Flux_d Lookup Table/1(Out1) -> psi_d/1, Product21/1(In1)
  psi_d/1 -> Product3/1(In1)
  Goto/1 -> From/1
  From/1 -> Lqq Lookup Table/1(In1), Ldd Lookup Table/1(In1)
  Ldd Lookup Table/1(Out1) -> Divide_recip/1(In1)
  From1/1 -> Lqq Lookup Table/2(In2), Ldd Lookup Table/2(In2)
  Goto1/1 -> From1/1
  Lqq Lookup Table/1(Out1) -> Divide1/2(In2)
  Switch1/1 -> Data Type Conversion17/1(In1)
  Data Type Conversion17/1(Out1) -> mux/4
  Data Type Conversion16/1(Out1) -> mux/3
  crp_out_delay5/1 -> Delay1_lowered1/1
  crp_out_delay4/1 -> Delay1_lowered2/1
  crp_out_delay3/1 -> Delay1/1
  crp_out_delay2/1 -> Delay/1
  crp_out_delay1/1 -> Delay1_lowered/1
  crp_out_delay/1 -> Delay11/1
  in3_repeat/1 -> delayMatch5/1
  Delay11/1 -> in3_repeat/1
  in4_repeat/1 -> delayMatch/1
  Delay1/1 -> in4_repeat/1
  in6_repeat/1 -> reset_out/3
  Delay1_lowered2/1 -> in6_repeat/1
  in7_repeat/1 -> reset_out1/3
  Delay1_lowered1/1 -> in7_repeat/1
  in9_repeat/1 -> delayMatch16/1
  Delay/1 -> in9_repeat/1
  in12_repeat/1 -> reset_out2/3
  Delay1_lowered/1 -> in12_repeat/1
  mux/1 -> t/1
  in13_repeat/1 -> Data Type Conversion10/1(In1)
  in11_repeat/1 -> Data Type Conversion13/1(In1)
  in10_repeat/1 -> t1/1
  in8_repeat/1 -> Data Type Conversion14/1(In1)
  in5_repeat/1 -> reset_out1/2, Rate Transition2/1, delayMatch18/1
  in2_repeat/1 -> Data Type Conversion6/1(In1)
  in1_repeat/1 -> delayMatch9/1, delayMatch12/1
  in0_repeat/1 -> Data Type Conversion12/1(In1)
  t/1 -> outputs/1
  inputs/1 -> in10_repeat/1
  psi_pm/1 -> psi_pm_term9/1
  polepairs/1 -> in13_repeat/1
  R1/1 -> in2_repeat/1
  reciprocal_L_q/1 -> reciprocal_L_q_term6/1
  reciprocal_L_d/1 -> reciprocal_L_d_term5/1
  M_n0/1 -> in11_repeat/1
  mu/1 -> in0_repeat/1
  reciprocal_J/1 -> in8_repeat/1
  simulate_mechanical/1 -> in1_repeat/1
  reset_integrators/1 -> in5_repeat/1

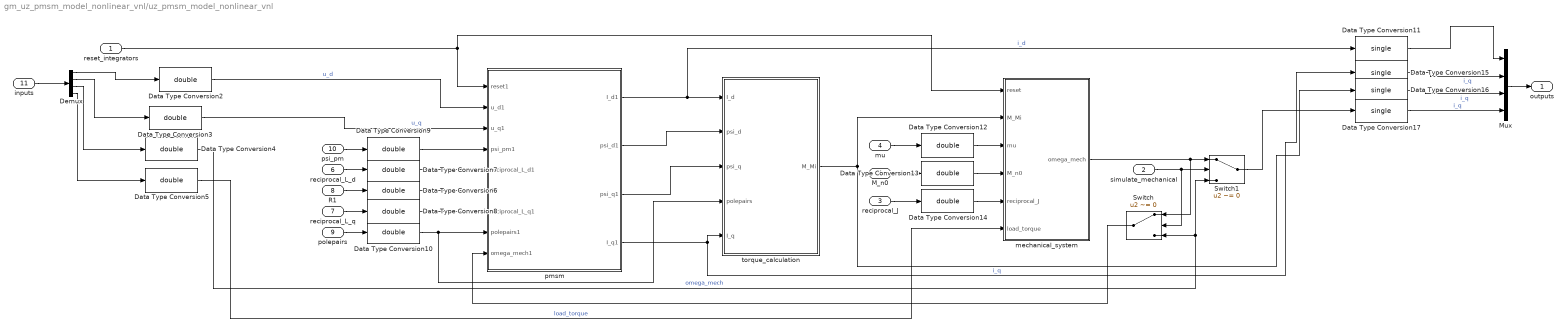
== system gm_uz_pmsm_model_nonlinear_vnl/uz_pmsm_model_nonlinear_vnl ==
  reset_integrators : Inport
  simulate_mechanical : Inport  Port=2
  reciprocal_J : Inport  Port=3
  mu : Inport  Port=4
  M_n0 : Inport  Port=5
  reciprocal_L_d : Inport  Port=6
  reciprocal_L_q : Inport  Port=7
  R1 : Inport  Port=8
  polepairs : Inport  Port=9
  psi_pm : Inport  Port=10
  inputs : Inport  Port=11
  Data Type Conversion{2..10,12..14} (12 alike) : DataTypeConversion  OutDataTypeStr=double  RndMeth=Nearest  SaturateOnIntegerOverflow=off
  Data Type Conversion{11,15..17} (4 alike) : DataTypeConversion  OutDataTypeStr=single  RndMeth=Nearest  SaturateOnIntegerOverflow=off
  Demux : Demux
  Mux : Mux
  Switch : Switch  Criteria=u2 ~= 0  SaturateOnIntegerOverflow=off  InputSameDT=off
  Switch1 : Switch  Criteria=u2 ~= 0  SaturateOnIntegerOverflow=off  InputSameDT=off
  mechanical_system : Subsystem
  pmsm : Subsystem
  torque_calculation : Subsystem
  outputs : Outport
  wires:
  Mux/1 -> outputs/1
  inputs/1 -> Demux/1
  Demux/4 -> Data Type Conversion5/1
  Demux/3 -> Data Type Conversion4/1
  Demux/2 -> Data Type Conversion3/1
  Demux/1 -> Data Type Conversion2/1
  Data Type Conversion11/1 -> Mux/1
  Data Type Conversion15/1 -> Mux/2  "i_q"
  Data Type Conversion16/1 -> Mux/3  "i_q"
  Data Type Conversion17/1 -> Mux/4  "i_q"
  pmsm/1(I_d1) -> torque_calculation/1(I_d), Data Type Conversion11/1  "i_d"
  pmsm/4(I_q1) -> Data Type Conversion15/1, torque_calculation/5(I_q)  "i_q"
  mechanical_system/1(omega_mech) -> Switch1/1, Switch/1
  Data Type Conversion3/1 -> pmsm/3(u_q1)  "u_q"
  polepairs/1 -> Data Type Conversion10/1
  reciprocal_L_q/1 -> Data Type Conversion8/1
  Data Type Conversion8/1 -> pmsm/7(reciprocal_L_q1)
  reciprocal_L_d/1 -> Data Type Conversion7/1
  Data Type Conversion13/1 -> mechanical_system/4(M_n0)
  psi_pm/1 -> Data Type Conversion9/1
  mu/1 -> Data Type Conversion12/1
  torque_calculation/1(M_Mi) -> Data Type Conversion16/1, mechanical_system/2(M_Mi)
  Data Type Conversion14/1 -> mechanical_system/5(reciprocal_J)
  M_n0/1 -> Data Type Conversion13/1
  simulate_mechanical/1 -> Switch/2, Switch1/2
  Data Type Conversion12/1 -> mechanical_system/3(mu)
  Data Type Conversion2/1 -> pmsm/2(u_d1)  "u_d"
  Data Type Conversion10/1 -> torque_calculation/4(polepairs), pmsm/8(polepairs1)
  pmsm/3(psi_q1) -> torque_calculation/3(psi_q)
  Data Type Conversion6/1 -> pmsm/6(R2)
  R1/1 -> Data Type Conversion6/1
  Data Type Conversion9/1 -> pmsm/4(psi_pm1)
  Switch1/1 -> Data Type Conversion17/1
  Data Type Conversion7/1 -> pmsm/5(reciprocal_L_d1)
  Data Type Conversion5/1 -> mechanical_system/6(load_torque)  "load_torque"
  pmsm/2(psi_d1) -> torque_calculation/2(psi_d)
  reciprocal_J/1 -> Data Type Conversion14/1
  Switch/1 -> pmsm/9(omega_mech1)
  Data Type Conversion4/1 -> Switch/3, Switch1/3  "omega_mech"
  reset_integrators/1 -> mechanical_system/1(reset), pmsm/1(reset1)

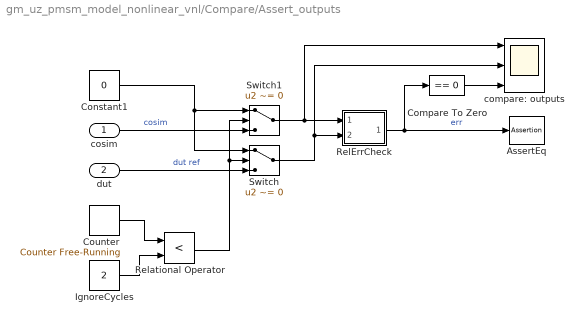
== system gm_uz_pmsm_model_nonlinear_vnl/Compare/Assert_outputs ==
  cosim : Inport
  dut : Inport  Port=2
  AssertEq : Assertion  StopWhenAssertionFail=off
  Compare To Zero : simulink/Logic and Bit Operations/Compare To Zero  relop===  OutDataTypeStr=boolean
  Constant1 : Constant  Value=0  OutDataTypeStr=Inherit: Inherit via back propagation  SampleTime=-1
  Counter : simulink/Sources/Counter Free-Running  NumBits=32  tsamp=-1
  IgnoreCycles : Constant  Value=2  OutDataTypeStr=Inherit: Inherit via back propagation  SampleTime=-1
  RelErrCheck : Subsystem
  Relational Operator : RelationalOperator  Operator=<  OutDataTypeStr=boolean  InputSameDT=off
  Switch : Switch  Criteria=u2 ~= 0  SaturateOnIntegerOverflow=off  InputSameDT=off
  Switch1 : Switch  Criteria=u2 ~= 0  SaturateOnIntegerOverflow=off  InputSameDT=off
  compare: outputs : Scope  NumInputPorts=3
  wires:
  IgnoreCycles/1 -> Relational Operator/2
  Counter/1 -> Relational Operator/1
  dut/1 -> Switch/3  "dut ref"
  cosim/1 -> Switch1/3  "cosim"
  Relational Operator/1 -> Switch1/2, Switch/2
  Constant1/1 -> Switch1/1, Switch/1
  Switch/1 -> compare: outputs/2, RelErrCheck/2(In2)
  Switch1/1 -> compare: outputs/1, RelErrCheck/1(In1)
  RelErrCheck/1(Out1) -> AssertEq/1, Compare To Zero/1  "err"
  Compare To Zero/1 -> compare: outputs/3

== system gm_uz_pmsm_model_nonlinear_vnl/Compare/CleanupScopes ==

== system gm_uz_pmsm_model_nonlinear_vnl/Compare/Enable ==

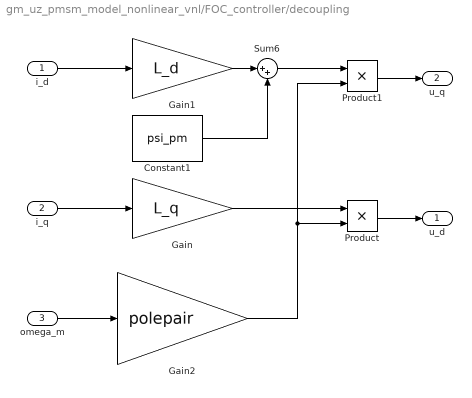
== system gm_uz_pmsm_model_nonlinear_vnl/FOC_controller/decoupling ==
  i_d : Inport
  i_q : Inport  Port=2
  omega_m : Inport  Port=3
  Constant1 : Constant  Value=psi_pm  SampleTime=-1
  Gain : Gain  Gain=L_q
  Gain1 : Gain  Gain=L_d
  Gain2 : Gain  Gain=polepair
  Product : Product
  Product1 : Product
  Sum6 : Sum  Inputs=|++
  u_d : Outport
  u_q : Outport  Port=2
  wires:
  Gain/1 -> Product/1
  Gain2/1 -> Product1/2, Product/2
  Product1/1 -> u_q/1
  i_d/1 -> Gain1/1
  Product/1 -> u_d/1
  Gain1/1 -> Sum6/1
  i_q/1 -> Gain/1
  Constant1/1 -> Sum6/2
  Sum6/1 -> Product1/1
  omega_m/1 -> Gain2/1

== system gm_uz_pmsm_model_nonlinear_vnl/uz_pmsm_model_nonlinear/Abs ==
  In1 : Inport
  Abs : Abs  SampleTime=1e-08  OutDataTypeStr=double  SaturateOnIntegerOverflow=off
  Out1 : Outport
  wires:
  Abs/1 -> Out1/1
  In1/1 -> Abs/1

== system gm_uz_pmsm_model_nonlinear_vnl/uz_pmsm_model_nonlinear/Data Type Conversion10 ==
  In1 : Inport
  Data Type Conversion10 : DataTypeConversion  OutDataTypeStr=double  RndMeth=Nearest  SampleTime=1e-08  SaturateOnIntegerOverflow=off
  Data Type Conversion10_pd1 : Delay  DelayLength=3
  Out1 : Outport
  wires:
  Data Type Conversion10_pd1/1 -> Out1/1
  Data Type Conversion10/1 -> Data Type Conversion10_pd1/1
  In1/1 -> Data Type Conversion10/1

== system gm_uz_pmsm_model_nonlinear_vnl/uz_pmsm_model_nonlinear/Data Type Conversion11 ==
  In1 : Inport
  Data Type Conversion11 : DataTypeConversion  OutDataTypeStr=single  RndMeth=Nearest  SampleTime=1e-08  SaturateOnIntegerOverflow=off
  Data Type Conversion11_pd1 : Delay  DelayLength=3
  Out1 : Outport
  wires:
  Data Type Conversion11_pd1/1 -> Out1/1
  Data Type Conversion11/1 -> Data Type Conversion11_pd1/1
  In1/1 -> Data Type Conversion11/1

== system gm_uz_pmsm_model_nonlinear_vnl/uz_pmsm_model_nonlinear/Data Type Conversion12 ==
  In1 : Inport
  Data Type Conversion12 : DataTypeConversion  OutDataTypeStr=double  RndMeth=Nearest  SampleTime=1e-08  SaturateOnIntegerOverflow=off
  Data Type Conversion12_pd1 : Delay  DelayLength=3
  Out1 : Outport
  wires:
  Data Type Conversion12_pd1/1 -> Out1/1
  Data Type Conversion12/1 -> Data Type Conversion12_pd1/1
  In1/1 -> Data Type Conversion12/1

== system gm_uz_pmsm_model_nonlinear_vnl/uz_pmsm_model_nonlinear/Data Type Conversion13 ==
  In1 : Inport
  Data Type Conversion13 : DataTypeConversion  OutDataTypeStr=double  RndMeth=Nearest  SampleTime=1e-08  SaturateOnIntegerOverflow=off
  Data Type Conversion13_pd1 : Delay  DelayLength=3
  Out1 : Outport
  wires:
  Data Type Conversion13_pd1/1 -> Out1/1
  Data Type Conversion13/1 -> Data Type Conversion13_pd1/1
  In1/1 -> Data Type Conversion13/1

== system gm_uz_pmsm_model_nonlinear_vnl/uz_pmsm_model_nonlinear/Data Type Conversion14 ==
  In1 : Inport
  Data Type Conversion14 : DataTypeConversion  OutDataTypeStr=double  RndMeth=Nearest  SampleTime=1e-08  SaturateOnIntegerOverflow=off
  Data Type Conversion14_pd1 : Delay  DelayLength=3
  Out1 : Outport
  wires:
  Data Type Conversion14_pd1/1 -> Out1/1
  Data Type Conversion14/1 -> Data Type Conversion14_pd1/1
  In1/1 -> Data Type Conversion14/1

== system gm_uz_pmsm_model_nonlinear_vnl/uz_pmsm_model_nonlinear/Data Type Conversion15 ==
  In1 : Inport
  Data Type Conversion15 : DataTypeConversion  OutDataTypeStr=single  RndMeth=Nearest  SampleTime=1e-08  SaturateOnIntegerOverflow=off
  Data Type Conversion15_pd1 : Delay  DelayLength=3
  Out1 : Outport
  wires:
  Data Type Conversion15_pd1/1 -> Out1/1
  Data Type Conversion15/1 -> Data Type Conversion15_pd1/1
  In1/1 -> Data Type Conversion15/1

== system gm_uz_pmsm_model_nonlinear_vnl/uz_pmsm_model_nonlinear/Data Type Conversion16 ==
  In1 : Inport
  Data Type Conversion16 : DataTypeConversion  OutDataTypeStr=single  RndMeth=Nearest  SampleTime=1e-08  SaturateOnIntegerOverflow=off
  Data Type Conversion16_pd1 : Delay  DelayLength=3
  Out1 : Outport
  wires:
  Data Type Conversion16_pd1/1 -> Out1/1
  Data Type Conversion16/1 -> Data Type Conversion16_pd1/1
  In1/1 -> Data Type Conversion16/1

== system gm_uz_pmsm_model_nonlinear_vnl/uz_pmsm_model_nonlinear/Data Type Conversion17 ==
  In1 : Inport
  Data Type Conversion17 : DataTypeConversion  OutDataTypeStr=single  RndMeth=Nearest  SampleTime=1e-08  SaturateOnIntegerOverflow=off
  Data Type Conversion17_pd1 : Delay  DelayLength=3
  Out1 : Outport
  wires:
  Data Type Conversion17_pd1/1 -> Out1/1
  Data Type Conversion17/1 -> Data Type Conversion17_pd1/1
  In1/1 -> Data Type Conversion17/1

== system gm_uz_pmsm_model_nonlinear_vnl/uz_pmsm_model_nonlinear/Data Type Conversion2 ==
  In1 : Inport
  Data Type Conversion2 : DataTypeConversion  OutDataTypeStr=double  RndMeth=Nearest  SampleTime=1e-08  SaturateOnIntegerOverflow=off
  Data Type Conversion2_pd1 : Delay  DelayLength=3
  Out1 : Outport
  wires:
  Data Type Conversion2_pd1/1 -> Out1/1
  Data Type Conversion2/1 -> Data Type Conversion2_pd1/1
  In1/1 -> Data Type Conversion2/1

== system gm_uz_pmsm_model_nonlinear_vnl/uz_pmsm_model_nonlinear/Data Type Conversion3 ==
  In1 : Inport
  Data Type Conversion3 : DataTypeConversion  OutDataTypeStr=double  RndMeth=Nearest  SampleTime=1e-08  SaturateOnIntegerOverflow=off
  Data Type Conversion3_pd1 : Delay  DelayLength=3
  Out1 : Outport
  wires:
  Data Type Conversion3_pd1/1 -> Out1/1
  Data Type Conversion3/1 -> Data Type Conversion3_pd1/1
  In1/1 -> Data Type Conversion3/1

== system gm_uz_pmsm_model_nonlinear_vnl/uz_pmsm_model_nonlinear/Data Type Conversion4 ==
  In1 : Inport
  Data Type Conversion4 : DataTypeConversion  OutDataTypeStr=double  RndMeth=Nearest  SampleTime=1e-08  SaturateOnIntegerOverflow=off
  Data Type Conversion4_pd1 : Delay  DelayLength=3
  Out1 : Outport
  wires:
  Data Type Conversion4_pd1/1 -> Out1/1
  Data Type Conversion4/1 -> Data Type Conversion4_pd1/1
  In1/1 -> Data Type Conversion4/1

== system gm_uz_pmsm_model_nonlinear_vnl/uz_pmsm_model_nonlinear/Data Type Conversion5 ==
  In1 : Inport
  Data Type Conversion5 : DataTypeConversion  OutDataTypeStr=double  RndMeth=Nearest  SampleTime=1e-08  SaturateOnIntegerOverflow=off
  Data Type Conversion5_pd1 : Delay  DelayLength=3
  Out1 : Outport
  wires:
  Data Type Conversion5_pd1/1 -> Out1/1
  Data Type Conversion5/1 -> Data Type Conversion5_pd1/1
  In1/1 -> Data Type Conversion5/1

== system gm_uz_pmsm_model_nonlinear_vnl/uz_pmsm_model_nonlinear/Data Type Conversion6 ==
  In1 : Inport
  Data Type Conversion6 : DataTypeConversion  OutDataTypeStr=double  RndMeth=Nearest  SampleTime=1e-08  SaturateOnIntegerOverflow=off
  Data Type Conversion6_pd1 : Delay  DelayLength=3
  Out1 : Outport
  wires:
  Data Type Conversion6_pd1/1 -> Out1/1
  Data Type Conversion6/1 -> Data Type Conversion6_pd1/1
  In1/1 -> Data Type Conversion6/1

== system gm_uz_pmsm_model_nonlinear_vnl/uz_pmsm_model_nonlinear/Divide ==
  In1 : Inport
  In2 : Inport  Port=2
  Divide : Product  Inputs=**  OutDataTypeStr=double  SampleTime=1e-08
  Divide_pd1 : Delay  DelayLength=6
  Out1 : Outport
  wires:
  Divide_pd1/1 -> Out1/1
  Divide/1 -> Divide_pd1/1
  In2/1 -> Divide/2
  In1/1 -> Divide/1

== system gm_uz_pmsm_model_nonlinear_vnl/uz_pmsm_model_nonlinear/Divide1 ==
  In1 : Inport
  In2 : Inport  Port=2
  Divide1 : Product  Inputs=*/  OutDataTypeStr=double  SampleTime=1e-08
  Divide1_pd1 : Delay  DelayLength=31
  Out1 : Outport
  wires:
  Divide1_pd1/1 -> Out1/1
  Divide1/1 -> Divide1_pd1/1
  In2/1 -> Divide1/2
  In1/1 -> Divide1/1
